simulink model "SF053A_HwAgVehCentrTrim"  (R2013b)
settings: Solver=FixedStepDiscrete  SolverMode=SingleTasking  StartTime=0.0  StopTime=1  FixedStep=0.002  RelTol=1e-3
values from neighbouring files (symbols this model uses):
  ENGRUNACTVTRUE_CNT_U08 = DataDict.Constant    [SF053A_HwAgVehCentrTrim_DataDict.m]
  HWAGCLRTRIMPRFMD_CNT_LGC = DataDict.Constant    [SF053A_HwAgVehCentrTrim_DataDict.m]
  HWAGCLRVAL_HWDEG_F32 = DataDict.Constant    [SF053A_HwAgVehCentrTrim_DataDict.m]
  HWAGEOTCCWNOTDETD_CNT_U08 = DataDict.Constant    [SF053A_HwAgVehCentrTrim_DataDict.m]
  HWAGEOTCWNOTDETD_CNT_U08 = DataDict.Constant    [SF053A_HwAgVehCentrTrim_DataDict.m]
  HWAGMAGTHDEXCDD_CNT_U08 = DataDict.Constant    [SF053A_HwAgVehCentrTrim_DataDict.m]
  HWAGTRIMPRFMD_CNT_LGC = DataDict.Constant    [SF053A_HwAgVehCentrTrim_DataDict.m]
  HwAgVehCentrTrimHwAgLim = DataDict.Calibration    [SF053A_HwAgVehCentrTrim_DataDict.m]
  HwAgVehCentrTrimVehSpdMaxThd = DataDict.Calibration    [SF053A_HwAgVehCentrTrim_DataDict.m]
  HwAgVehCentrTrimVld = DataDict.NTC    [SF053A_HwAgVehCentrTrim_DataDict.m]
  NODEBSTEP_CNT_U16 = DataDict.Constant    [SF053A_HwAgVehCentrTrim_DataDict.m]
  UPDHWAGTRIMPRFMD_CNT_U08 = DataDict.Constant    [SF053A_HwAgVehCentrTrim_DataDict.m]
  VEHSPDTHDEXCDD_CNT_U08 = DataDict.Constant    [SF053A_HwAgVehCentrTrim_DataDict.m]
undefined symbols (not defined in the file or in its folder): NtcSts1, u2, u3, u4, u5
libraries: simulink x6, NxtrNvM x3, NxtrLim x2
(part 3 of 3)

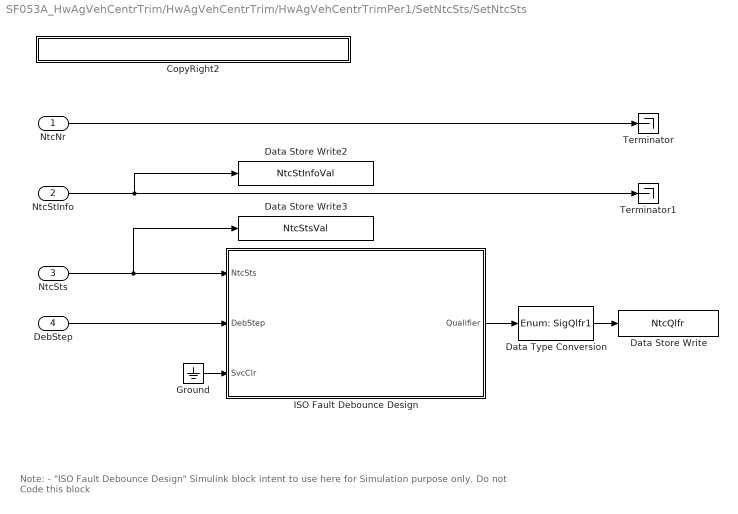
== system SF053A_HwAgVehCentrTrim/HwAgVehCentrTrim/HwAgVehCentrTrimPer1/SetNtcSts/SetNtcSts ==
  note: Note:
      |
      | - "ISO Fault Debounce Design" Simulink block intent to use here for Simulation purpose only. Do not Code this block
  NtcNr : Inport
  NtcStInfo : Inport  Port=2
  NtcSts : Inport  Port=3
  DebStep : Inport  Port=4
  CopyRight2 : Subsystem  Description=|  mask(Copyright Information){none=on}
      | Copyright info block.                                               
      |                                                                     
      | Place copyright information at the top of every subsystem in design.
      mask prompts: none "No parameters"
      mask help: Place copyright information at the top of every subsystem in design.
      mask Display:
      | NxtrConf = 'Nexteer Confidential';
      | 
      | sys = bdroot; %handle for the current model ("system")
      | first = get_param(sys,'Created');
      | first = first(end-3:end);  %year is last four digits
      | 
      | last = get_param(sys,'LastModifiedDate');
      | if isempty(last)
      |     last = datestr(now,'yyyy');
      | else
      |     last = last(end-3:end);
      | end
      | 
      | if strcmp(first,last)
      |     fprintf('%s -- Copyright %s Nexteer',NxtrConf,first)
      | else
      |     fprintf('%s -- %s%s- %s Nexteer',NxtrConf,char(169),first,last)
      | end
  Data Store Write : DataStoreWrite  DataStoreName=NtcQlfr
  Data Store Write2 : DataStoreWrite  DataStoreName=NtcStInfoVal
  Data Store Write3 : DataStoreWrite  DataStoreName=NtcStsVal
  Data Type Conversion : DataTypeConversion  OutDataTypeStr=Enum: SigQlfr1
  Ground : Ground
  ISO Fault Debounce Design : Stateflow chart  TreatAsAtomicUnit=on
      settings: AttributesFormatString=|
      | Simulation Purpose Only.
      | Do Not Code this block
      | Diagnostic Manager Owns this requirement
  Terminator : Terminator
  Terminator1 : Terminator
  wires:
  NtcStInfo/1 -> Data Store Write2/1, Terminator1/1
  NtcNr/1 -> Terminator/1
  NtcSts/1 -> Data Store Write3/1, ISO Fault Debounce Design/1(NtcSts)
  DebStep/1 -> ISO Fault Debounce Design/2(DebStep)
  ISO Fault Debounce Design/1(Qualifier) -> Data Type Conversion/1
  Ground/1 -> ISO Fault Debounce Design/3(SvcClr)
  Data Type Conversion/1 -> Data Store Write/1

== system SF053A_HwAgVehCentrTrim/HwAgVehCentrTrim/UpdHwAgTrimVal/EngRunActvTrue/CopyRight2 ==

== system SF053A_HwAgVehCentrTrim/HwAgVehCentrTrim/UpdHwAgTrimVal/HwAgEotCcwNotDetd/CopyRight2 ==

== system SF053A_HwAgVehCentrTrim/HwAgVehCentrTrim/UpdHwAgTrimVal/HwAgEotCwNotDetd/CopyRight2 ==

== system SF053A_HwAgVehCentrTrim/HwAgVehCentrTrim/UpdHwAgTrimVal/HwAgMagThdExcdd/CopyRight2 ==

== system SF053A_HwAgVehCentrTrim/HwAgVehCentrTrim/UpdHwAgTrimVal/SetNtcSts/CopyRight2 ==

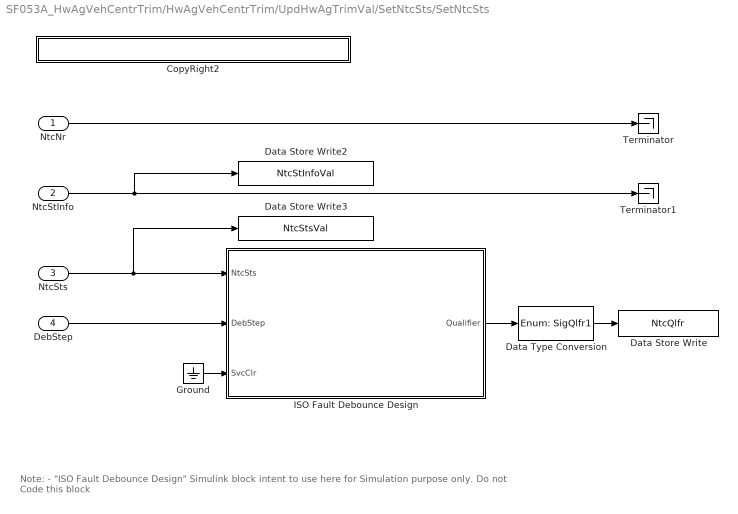
== system SF053A_HwAgVehCentrTrim/HwAgVehCentrTrim/UpdHwAgTrimVal/SetNtcSts/SetNtcSts ==
  note: Note:
      |
      | - "ISO Fault Debounce Design" Simulink block intent to use here for Simulation purpose only. Do not Code this block
  NtcNr : Inport
  NtcStInfo : Inport  Port=2
  NtcSts : Inport  Port=3
  DebStep : Inport  Port=4
  CopyRight2 : Subsystem  Description=|  mask(Copyright Information){none=on}
      | Copyright info block.                                               
      |                                                                     
      | Place copyright information at the top of every subsystem in design.
      mask prompts: none "No parameters"
      mask help: Place copyright information at the top of every subsystem in design.
      mask Display:
      | NxtrConf = 'Nexteer Confidential';
      | 
      | sys = bdroot; %handle for the current model ("system")
      | first = get_param(sys,'Created');
      | first = first(end-3:end);  %year is last four digits
      | 
      | last = get_param(sys,'LastModifiedDate');
      | if isempty(last)
      |     last = datestr(now,'yyyy');
      | else
      |     last = last(end-3:end);
      | end
      | 
      | if strcmp(first,last)
      |     fprintf('%s -- Copyright %s Nexteer',NxtrConf,first)
      | else
      |     fprintf('%s -- %s%s- %s Nexteer',NxtrConf,char(169),first,last)
      | end
  Data Store Write : DataStoreWrite  DataStoreName=NtcQlfr
  Data Store Write2 : DataStoreWrite  DataStoreName=NtcStInfoVal
  Data Store Write3 : DataStoreWrite  DataStoreName=NtcStsVal
  Data Type Conversion : DataTypeConversion  OutDataTypeStr=Enum: SigQlfr1
  Ground : Ground
  ISO Fault Debounce Design : Stateflow chart  TreatAsAtomicUnit=on
      settings: AttributesFormatString=|
      | Simulation Purpose Only.
      | Do Not Code this block
      | Diagnostic Manager Owns this requirement
  Terminator : Terminator
  Terminator1 : Terminator
  wires:
  NtcStInfo/1 -> Data Store Write2/1, Terminator1/1
  NtcNr/1 -> Terminator/1
  NtcSts/1 -> Data Store Write3/1, ISO Fault Debounce Design/1(NtcSts)
  DebStep/1 -> ISO Fault Debounce Design/2(DebStep)
  ISO Fault Debounce Design/1(Qualifier) -> Data Type Conversion/1
  Ground/1 -> ISO Fault Debounce Design/3(SvcClr)
  Data Type Conversion/1 -> Data Store Write/1

== system SF053A_HwAgVehCentrTrim/HwAgVehCentrTrim/UpdHwAgTrimVal/SetNtcSts1/CopyRight2 ==

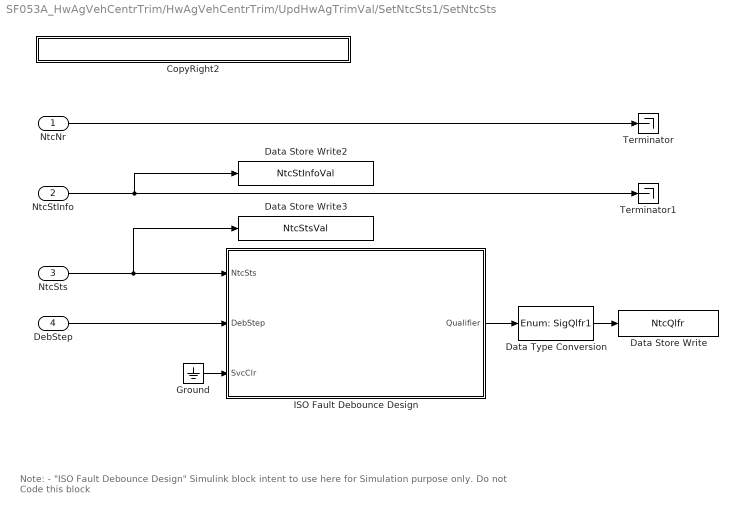
== system SF053A_HwAgVehCentrTrim/HwAgVehCentrTrim/UpdHwAgTrimVal/SetNtcSts1/SetNtcSts ==
  note: Note:
      |
      | - "ISO Fault Debounce Design" Simulink block intent to use here for Simulation purpose only. Do not Code this block
  NtcNr : Inport
  NtcStInfo : Inport  Port=2
  NtcSts : Inport  Port=3
  DebStep : Inport  Port=4
  CopyRight2 : Subsystem  Description=|  mask(Copyright Information){none=on}
      | Copyright info block.                                               
      |                                                                     
      | Place copyright information at the top of every subsystem in design.
      mask prompts: none "No parameters"
      mask help: Place copyright information at the top of every subsystem in design.
      mask Display:
      | NxtrConf = 'Nexteer Confidential';
      | 
      | sys = bdroot; %handle for the current model ("system")
      | first = get_param(sys,'Created');
      | first = first(end-3:end);  %year is last four digits
      | 
      | last = get_param(sys,'LastModifiedDate');
      | if isempty(last)
      |     last = datestr(now,'yyyy');
      | else
      |     last = last(end-3:end);
      | end
      | 
      | if strcmp(first,last)
      |     fprintf('%s -- Copyright %s Nexteer',NxtrConf,first)
      | else
      |     fprintf('%s -- %s%s- %s Nexteer',NxtrConf,char(169),first,last)
      | end
  Data Store Write : DataStoreWrite  DataStoreName=NtcQlfr
  Data Store Write2 : DataStoreWrite  DataStoreName=NtcStInfoVal
  Data Store Write3 : DataStoreWrite  DataStoreName=NtcStsVal
  Data Type Conversion : DataTypeConversion  OutDataTypeStr=Enum: SigQlfr1
  Ground : Ground
  ISO Fault Debounce Design : Stateflow chart  TreatAsAtomicUnit=on
      settings: AttributesFormatString=|
      | Simulation Purpose Only.
      | Do Not Code this block
      | Diagnostic Manager Owns this requirement
  Terminator : Terminator
  Terminator1 : Terminator
  wires:
  NtcStInfo/1 -> Data Store Write2/1, Terminator1/1
  NtcNr/1 -> Terminator/1
  NtcSts/1 -> Data Store Write3/1, ISO Fault Debounce Design/1(NtcSts)
  DebStep/1 -> ISO Fault Debounce Design/2(DebStep)
  ISO Fault Debounce Design/1(Qualifier) -> Data Type Conversion/1
  Ground/1 -> ISO Fault Debounce Design/3(SvcClr)
  Data Type Conversion/1 -> Data Store Write/1

== system SF053A_HwAgVehCentrTrim/HwAgVehCentrTrim/UpdHwAgTrimVal/UpdHwAgTrimPrfmd/CopyRight2 ==

== system SF053A_HwAgVehCentrTrim/HwAgVehCentrTrim/UpdHwAgTrimVal/VehSpdThdExcdd/CopyRight2 ==

== system SF053A_HwAgVehCentrTrim/HwAgVehCentrTrim/HwAgVehCentrTrimInit1/SetNtcSts/SetNtcSts/CopyRight2 ==

== system SF053A_HwAgVehCentrTrim/HwAgVehCentrTrim/HwAgVehCentrTrimPer1/SetNtcSts/SetNtcSts/CopyRight2 ==

== system SF053A_HwAgVehCentrTrim/HwAgVehCentrTrim/UpdHwAgTrimVal/SetNtcSts/SetNtcSts/CopyRight2 ==

== system SF053A_HwAgVehCentrTrim/HwAgVehCentrTrim/UpdHwAgTrimVal/SetNtcSts1/SetNtcSts/CopyRight2 ==
